simulink model "SignalVirtual"  (R2017b)
settings: Solver=FixedStepAuto  StartTime=0.0  StopTime=10.0  FixedStep=1.000000  RelTol=1e-3  EnableMultiTasking=on
PreLoadFcn:
  | % Bus object: subBus
  | clear elems;
  | elems(1) = Simulink.BusElement;
  | elems(1).Name = 'chirp';
  | elems(1).Dimensions = 1;
  | elems(1).DimensionsMode = 'Fixed';
  | elems(1).DataType = 'double';
  | elems(1).SampleTime = -1;
  | elems(1).Complexity = 'real';
  | elems(1).Min = [];
  | elems(1).Max = [];
  | elems(1).DocUnits = '';
  | elems(1).Description = '';
  | 
  | elems(2) = Simulink.BusElement;
  | elems(2).Name = 'sine';
  | elems(2).Dimensions = 1;
  | elems(2).DimensionsMode = 'Fixed';
  | elems(2).DataType = 'double';
  | elems(2).SampleTime = -1;
  | elems(2).Complexity = 'real';
  | elems(2).Min = [];
  | elems(2).Max = [];
  | elems(2).DocUnits = '';
  | elems(2).Description = '';
  | 
  | subBus = Simulink.Bus;
  | subBus.HeaderFile = '';
  | subBus.Description = '';
  | subBus.DataScope = 'Auto';
  | subBus.Alignment = -1;
  | subBus.Elements = elems;
  | clear elems;
  | assignin('base','subBus', subBus);
settings Model: Creator=arnaud  LastModifiedBy=hbourbou
settings DataIOCC: LimitDataPoints=on  SaveFormat=StructureWithTime  SignalLoggingSaveFormat=ModelDataLogs
settings OptimizationCC: ExpressionDepthLimit=2147483647  LifeSpan=inf
settings DebuggingCC: UnderspecifiedInitializationDetection=Classic  MergeDetectMultiDrivingBlocksExec=none  SolverPrmCheckMsg=warning  FcnCallInpInsideContextMsg=warning  StateNameClashWarn=warning  SFUnexpectedBacktrackingDiag=warning  SFNoUnconditionalDefaultTransitionDiag=warning  SFExecutionAtInitializationDiag=none
settings HardwareCC: ProdBitPerPointer=32  ProdBitPerSizeT=32  ProdBitPerPtrDiffT=32  ProdLargestAtomicFloat=None  ProdIntDivRoundTo=Undefined  ProdEndianess=Unspecified  ProdWordSize=32  ProdHWDeviceType=32-bit Generic
settings ModelReferenceCC: PropagateSignalLabelsOutOfModel=off
settings CodeAppCC: StateflowObjectComments=on
settings GRTTargetCC: TargetLangStandard=C89/C90 (ANSI)  GeneratePreprocessorConditionals=Disable all  CombineOutputUpdateFcns=off  GRTInterface=on
settings ConfigComp: CovMetricSettings=dw  CovHtmlReporting=on  CovSaveCumulativeToWorkspaceVar=on  CovSaveSingleToWorkspaceVar=on  CovExternalEMLEnable=off  CovSFcnEnable=off

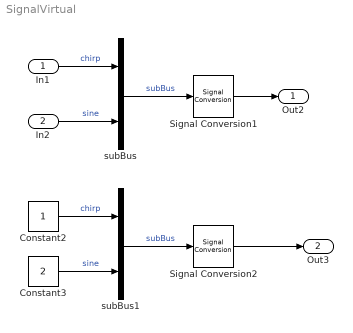
== system SignalVirtual ==
  In1 : Inport  OutDataTypeStr=double  PortDimensions=1
  In2 : Inport  Port=2  OutDataTypeStr=double  PortDimensions=1
  Constant2 : Constant
  Constant3 : Constant  Value=2
  Signal Conversion1 : SignalConversion  ConversionOutput=Virtual bus  OverrideOpt=off
  Signal Conversion2 : SignalConversion  ConversionOutput=Virtual bus  OverrideOpt=off
  subBus : BusCreator  Inputs=2
  subBus1 : BusCreator  Inputs=2  OutDataTypeStr=Bus: subBus  NonVirtualBus=on
  Out2 : Outport
  Out3 : Outport  Port=2
  wires:
  In1/1 -> subBus/1  "chirp"
  In2/1 -> subBus/2  "sine"
  subBus/1 -> Signal Conversion1/1  "subBus"
  Signal Conversion1/1 -> Out2/1
  Signal Conversion2/1 -> Out3/1
  Constant2/1 -> subBus1/1  "chirp"
  Constant3/1 -> subBus1/2  "sine"
  subBus1/1 -> Signal Conversion2/1  "subBus"
